simulink model "RPkiAux1"  (R2020a)
settings: Solver=ode45  StartTime=0.0  StopTime=8  MaxStep=1e-3  RelTol=1e-6  AbsTol=1e-6
InitFcn:
  | k = 0.9;
  | m = 1.5;
  | l = 1;
  | g = 9.81;
  | 
  | phi0a = 3*pi/4 - 2*pi;
  | om0a = 15;
  | phi0b = -pi;
  | om0b = sqrt(g/l);
  | phi0c = -3*pi;
  | om0c = sqrt(g/l);
  | phi0d = -5*pi;
  | om0d = sqrt(g/l);
  | 
  | phi0 = phi0d;
  | om0 = om0d;
libraries: simulink x1
settings Model: Creator=Home  LastModifiedBy=peter

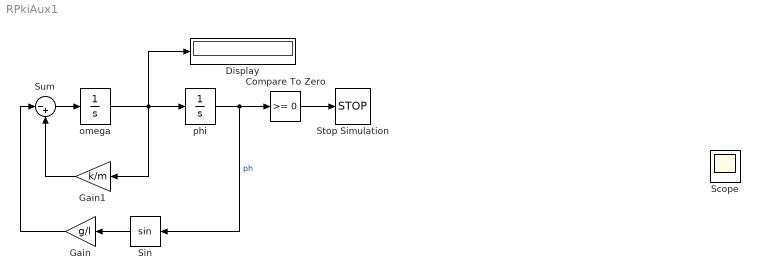
== system RPkiAux1 ==
  Compare To Zero : simulink/Logic and Bit Operations/Compare To Zero  relop=>=  OutDataTypeStr=boolean
  Display : Display
  Gain : Gain  Gain=g/l
  Gain1 : Gain  Gain=k/m
  Sin : Trigonometry
  Stop Simulation : Stop
  Sum : Sum  Inputs=|-+
  omega : Integrator  InitialCondition=om0
  phi : Integrator  InitialCondition=phi0
  Scope : Scope
  wires:
  phi/1 -> Compare To Zero/1, Sin/1  "ph"
  Sin/1 -> Gain/1
  Sum/1 -> omega/1
  omega/1 -> Display/1, Gain1/1, phi/1
  Gain1/1 -> Sum/2
  Gain/1 -> Sum/1
  Compare To Zero/1 -> Stop Simulation/1
